simulink model "motor_model_ss"  (R2015a)
settings: Solver=ode45  StartTime=0.0  StopTime=10.0  RelTol=1e-3
values from neighbouring files (symbols this model uses):
  C1 = 0.9*9.81    (= 8.829)    [Sim_SS.m]
  C2 = 0.5*1.225*(0.10)^2*1.05    (= 0.00643125)    [Sim_SS.m]
  Kf = 0.26    [Sim.m]    (also in Sim_SS.m = 0.2625)
  M = 1    [Sim.m]    (also in Sim_SS.m = 1.5)
  NM = 2    [Sim.m]    (also in Sim_SS.m)
  R = 0.03    [Sim.m]    (also in Sim_SS.m)
  Ra = 5.625    [Sim.m]    (also in Sim_SS.m = 0.0712)
  theta = 5*pi/180    (= 0.0872664625997)    [Sim.m]    (also in Sim_SS.m)
  Ua = 4.5    [Sim_SS.m]
libraries: simulink x1
settings Model: Creator=Paul  LastModifiedBy=miguel

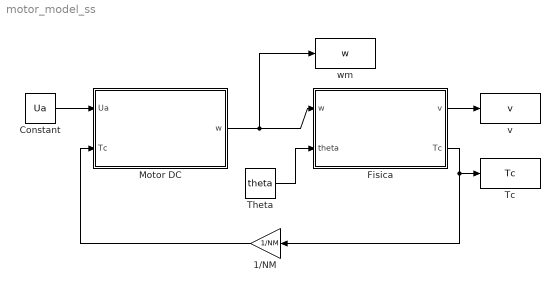
== system motor_model_ss ==
  1/NM : Gain  Gain=1/NM
  Constant : Constant  Value=Ua
  Fisica : Subsystem
  Motor DC : Subsystem
  Tc : ToWorkspace  VariableName=Tc  SampleTime=-1
  Theta : Constant  Value=theta
  v : ToWorkspace  VariableName=v  SampleTime=-1
  wm : ToWorkspace  VariableName=w  SampleTime=-1
  wires:
  Motor DC/1(w) -> wm/1, Fisica/1(w)
  Fisica/1(v) -> v/1
  Fisica/2(Tc) -> Tc/1, 1/NM/1
  1/NM/1 -> Motor DC/2(Tc)
  Constant/1 -> Motor DC/1("Ua ")
  Theta/1 -> Fisica/2(theta)

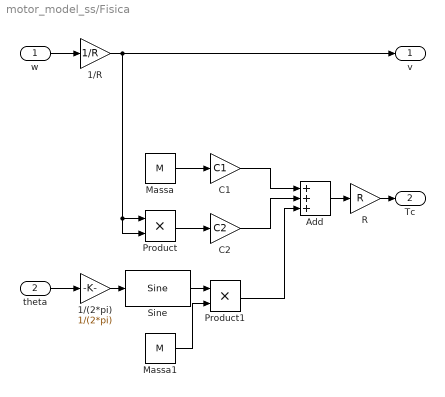
== system motor_model_ss/Fisica ==
  w : Inport
  theta : Inport  Port=2
  1/(2*pi) : Gain  Gain=1/(2*pi)
  1/R : Gain  Gain=1/R
  Add : Sum  Inputs=+++
  C1 : Gain  Gain=C1
  C2 : Gain  Gain=C2
  Massa : Constant  Value=M
  Massa1 : Constant  Value=M
  Product : Product
  Product1 : Product
  R : Gain  Gain=R
  Sine : simulink/Lookup Tables/Sine  Formula=sin(2*pi*u)  NumDataPoints=(2^5)+1  OutputWordLength=16  InternalRulePriority=Speed
  v : Outport
  Tc : Outport  Port=2
  wires:
  1/R/1 -> Product/1, Product/2, v/1
  w/1 -> 1/R/1
  R/1 -> Tc/1
  Add/1 -> R/1
  Product/1 -> C2/1
  C2/1 -> Add/2
  Massa/1 -> C1/1
  C1/1 -> Add/1
  Massa1/1 -> Product1/2
  Product1/1 -> Add/3
  Sine/1 -> Product1/1
  1/(2*pi)/1 -> Sine/1
  theta/1 -> 1/(2*pi)/1

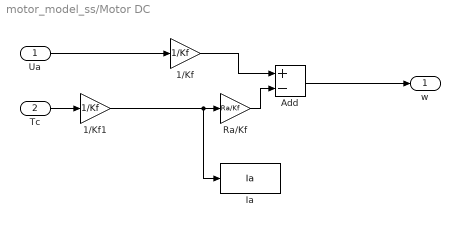
== system motor_model_ss/Motor DC ==
  "Ua " : Inport
  Tc : Inport  Port=2
  1/Kf : Gain  Gain=1/Kf
  1/Kf1 : Gain  Gain=1/Kf
  Add : Sum  Inputs=+-
  Ia : ToWorkspace  VariableName=Ia  SampleTime=-1
  Ra/Kf : Gain  Gain=Ra/Kf
  w : Outport
  wires:
  "Ua "/1 -> 1/Kf/1
  1/Kf/1 -> Add/1
  Ra/Kf/1 -> Add/2
  Add/1 -> w/1
  Tc/1 -> 1/Kf1/1
  1/Kf1/1 -> Ra/Kf/1, Ia/1
